simulink model "Prvi"  (R2020a)
settings: Solver=VariableStepAuto  StartTime=0.0  StopTime=20  RelTol=1e-3
settings Model: Creator=Emina  LastModifiedBy=Aldin

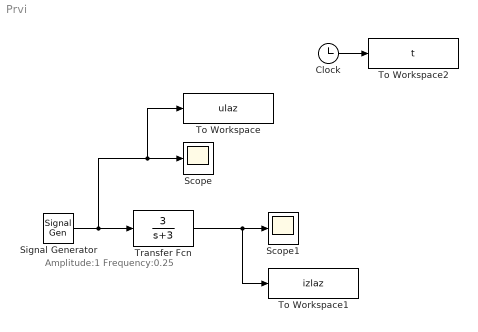
== system Prvi ==
  note: Amplitude:1
      | Frequency:0.25
  Clock : Clock
  Scope : Scope
  Scope1 : Scope
  Signal Generator : SignalGenerator  WaveForm=square  Frequency=0.25
  To Workspace : ToWorkspace  VariableName=ulaz  SampleTime=-1
  To Workspace1 : ToWorkspace  VariableName=izlaz  SampleTime=-1
  To Workspace2 : ToWorkspace  VariableName=t  SampleTime=-1
  Transfer Fcn : TransferFcn  Numerator=[3]  Denominator=[1 3]
  wires:
  Signal Generator/1 -> To Workspace/1, Scope/1, Transfer Fcn/1
  Transfer Fcn/1 -> To Workspace1/1, Scope1/1
  Clock/1 -> To Workspace2/1
